simulink model "ThrottlePositionSensor"  (R2023a)
settings: Solver=FixedStepAuto  StartTime=0.0  StopTime=10.0  RelTol=1e-3
undefined symbols (not defined in the file or in its folder): TPS_Modes
libraries: pil_lib x1
settings Model: Creator=EMRIX  LastModifiedBy=EMRIX
settings OptimizationCC: DefaultParameterBehavior=Inlined  UseDivisionForNetSlopeComputation=on  GainParamInheritBuiltInType=on  UseFloatMulNetSlope=on  InlineInvariantSignals=on  PassReuseOutputArgsAs=Individual arguments  ZeroExternalMemoryAtStartup=off  ZeroInternalMemoryAtStartup=off  NoFixptDivByZeroProtection=on  EfficientFloat2IntCast=on  LifeSpan=1  OptimizeBlockOrder=speed  DifferentSizesBufferReuse=on  EfficientTunableParamExpr=on
settings DebuggingCC: ParameterTunabilityLossMsg=error
settings HardwareCC: ProdLongLongMode=on
settings SFSimCC: MATLABDynamicMemAlloc=off
settings RTWCC: Description=Embedded Coder  SystemTargetFile=ert.tlc  TemplateMakefile=ert_default_tmf  CreateSILPILBlock=SIL
settings CodeAppCC: ForceParamTrailComments=on  IgnoreCustomStorageClasses=off  OperatorAnnotations=on  SimulinkDataObjDesc=on  SFDataObjDesc=on  CustomSymbolStrGlobalVar=rt$N$M  CustomSymbolStrType=$N$M  CustomSymbolStrFcn=$N$M$F  CustomSymbolStrMacro=$N$M  InsertBlockDesc=on
settings ERTTargetCC: TargetLangStandard=C99 (ISO)  GenerateSampleERTMain=on  IncludeMdlTerminateFcn=off  CombineSignalStateStructs=on  SuppressErrorStatus=on  SupportAbsoluteTime=off  SupportComplex=off  InlinedParameterPlacement=NonHierarchical  ERTCustomFileTemplate=example_file_process.tlc  ERTFilePackagingFormat=CompactWithDataFile

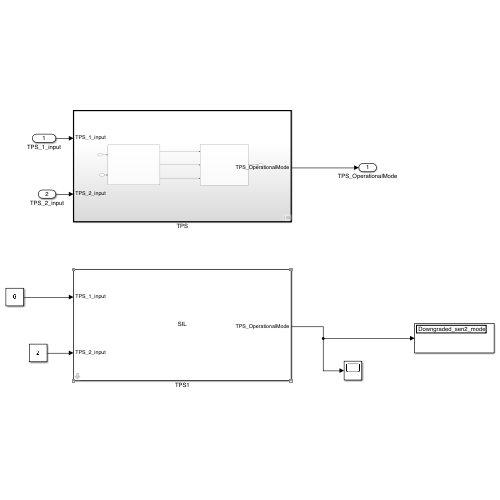
[thumbnail: Simulink's stored preview of the top-level diagram]
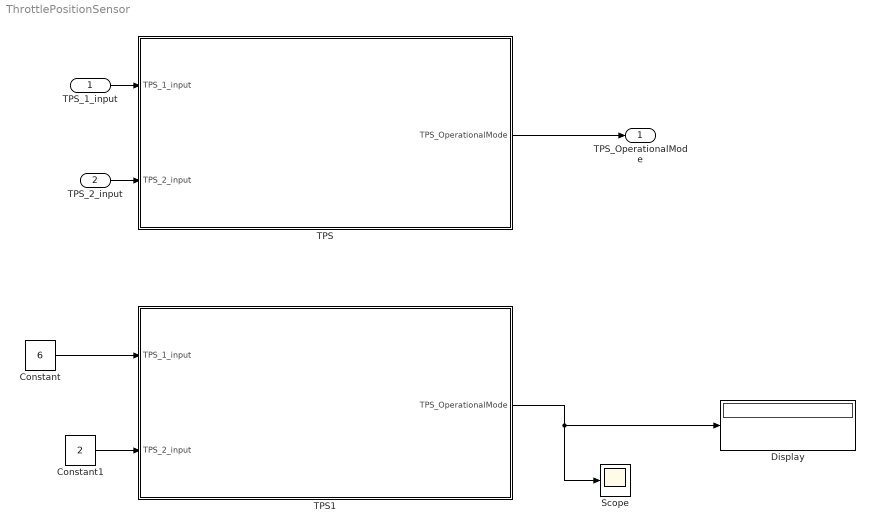
== system ThrottlePositionSensor ==
  TPS_1_input : Inport
  TPS_2_input : Inport  Port=2
  Constant : Constant  Value=6  OutDataTypeStr=Inherit: Inherit via back propagation
  Constant1 : Constant  Value=2  OutDataTypeStr=Inherit: Inherit via back propagation
  Display : Display
  Scope : Scope
  TPS : Subsystem  TreatAsAtomicUnit=on
  TPS1 : Subsystem  Tag=__SL_testing_harness_stub_  DialogController=pil_create_dialog  LoadFcn=|
      | try
      |    if ~strcmp(rtw.pil.getPILVersion, '9.14 (R2023a)_15')
      |       set_param(gcb, 'DialogController', '');
      |       set_param(gcb, 'DialogControllerArgs', '');
      |    end
      | catch e
      |       set_param(gcb, 'DialogController', '');
      |       set_param(gcb, 'DialogControllerArgs', '');
      | end
      mask help: PIL:pil:XILBlockMaskDesc
      mask Display: disp('SIL');
  TPS_OperationalMode : Outport
  wires:
  TPS/1(TPS_OperationalMode) -> TPS_OperationalMode/1
  TPS_2_input/1 -> TPS/2(TPS_2_input)
  TPS_1_input/1 -> TPS/1(TPS_1_input)
  Constant1/1 -> TPS1/2(TPS_2_input)
  Constant/1 -> TPS1/1(TPS_1_input)
  TPS1/1(TPS_OperationalMode) -> Scope/1, Display/1

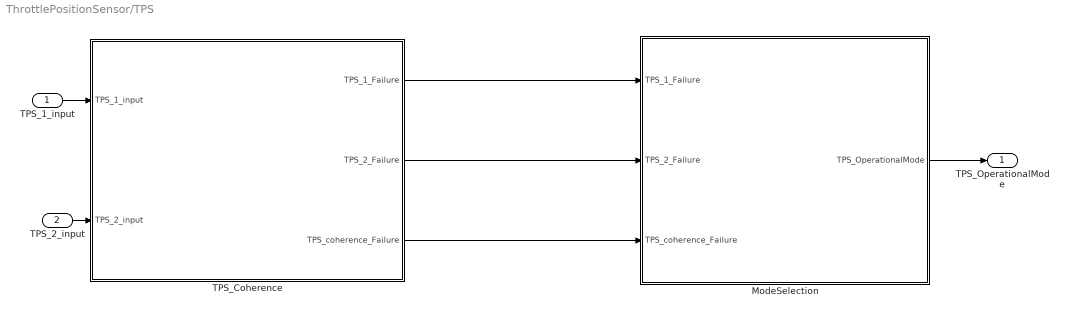
== system ThrottlePositionSensor/TPS ==
  TPS_1_input : Inport  OutDataTypeStr=single
  TPS_2_input : Inport  Port=2  OutDataTypeStr=single
  ModeSelection : Subsystem
  TPS_Coherence : Subsystem
      mask DialogControl TPS_Coherence Prompt: Parameters
  TPS_OperationalMode : Outport
  wires:
  TPS_2_input/1 -> TPS_Coherence/2(TPS_2_input)
  TPS_1_input/1 -> TPS_Coherence/1(TPS_1_input)
  ModeSelection/1(TPS_OperationalMode) -> TPS_OperationalMode/1
  TPS_Coherence/1(TPS_1_Failure) -> ModeSelection/1(TPS_1_Failure)
  TPS_Coherence/2(TPS_2_Failure) -> ModeSelection/2(TPS_2_Failure)
  TPS_Coherence/3(TPS_coherence_Failure) -> ModeSelection/3(TPS_coherence_Failure)

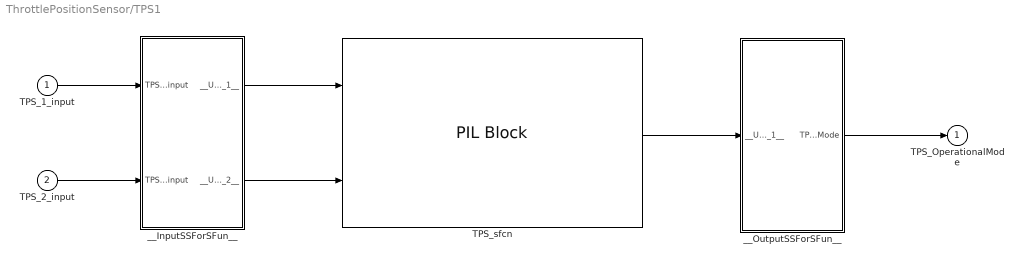
== system ThrottlePositionSensor/TPS1 ==
  TPS_1_input : Inport  OutDataTypeStr=single
  TPS_2_input : Inport  Port=2  OutDataTypeStr=single
  TPS_sfcn : pil_lib/PIL Block  SimulationMode=SIL  IsTopModelPIL=off  CodeDir=TPS_ert_rtw  AnchorDir=F:\XELLED\OS-Academy MBD\Labs\SimuLink Labs\System_Modelling_Module\TPS  ConfigName=Software-in-the-Loop (SIL)  XrelIsTopModelCode=on  XrelIsReusable=off  XrelDWorkNames={}  XrelDWorkTypes={}  XrelModelArgVals={}  XrelOrderedParamNames={}
  __InputSSForSFun__ : Subsystem
  __OutputSSForSFun__ : Subsystem
  TPS_OperationalMode : Outport
  wires:
  __OutputSSForSFun__/1(TPS_OperationalMode) -> TPS_OperationalMode/1
  TPS_sfcn/1 -> __OutputSSForSFun__/1(__UniqueInportName__1__)
  __InputSSForSFun__/2(__UniqueOutportName__2__) -> TPS_sfcn/2
  __InputSSForSFun__/1(__UniqueOutportName__1__) -> TPS_sfcn/1
  TPS_2_input/1 -> __InputSSForSFun__/2(TPS_2_input)
  TPS_1_input/1 -> __InputSSForSFun__/1(TPS_1_input)

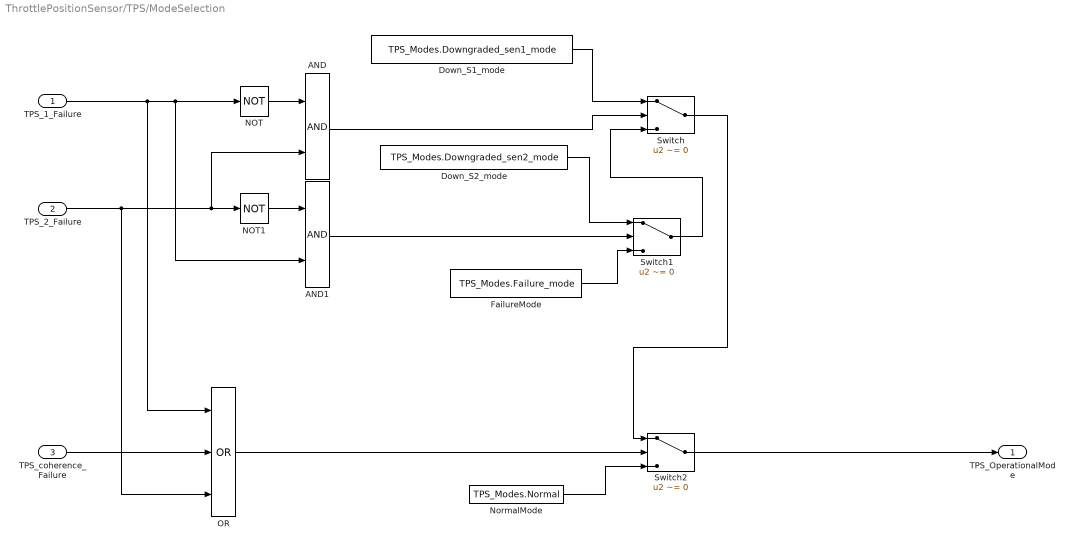
== system ThrottlePositionSensor/TPS/ModeSelection ==
  TPS_1_Failure : Inport  OutDataTypeStr=boolean
  TPS_2_Failure : Inport  Port=2  OutDataTypeStr=boolean
  TPS_coherence_Failure : Inport  Port=3  OutDataTypeStr=boolean
  AND : Logic  AllPortsSameDT=off  OutDataTypeStr=boolean
  AND1 : Logic  AllPortsSameDT=off  OutDataTypeStr=boolean
  Down_S1_mode : Constant  Value=TPS_Modes.Downgraded_sen1_mode
  Down_S2_mode : Constant  Value=TPS_Modes.Downgraded_sen2_mode
  FailureMode : Constant  Value=TPS_Modes.Failure_mode
  NOT : Logic  Operator=NOT  AllPortsSameDT=off  OutDataTypeStr=boolean
  NOT1 : Logic  Operator=NOT  AllPortsSameDT=off  OutDataTypeStr=boolean
  NormalMode : Constant  Value=TPS_Modes.Normal
  OR : Logic  Operator=OR  Inputs=3  AllPortsSameDT=off  OutDataTypeStr=boolean
  Switch : Switch  Criteria=u2 ~= 0  SaturateOnIntegerOverflow=off  InputSameDT=off
  Switch1 : Switch  Criteria=u2 ~= 0  SaturateOnIntegerOverflow=off  InputSameDT=off
  Switch2 : Switch  Criteria=u2 ~= 0  SaturateOnIntegerOverflow=off  InputSameDT=off
  TPS_OperationalMode : Outport
  wires:
  NOT/1 -> AND/1
  AND/1 -> Switch/2
  TPS_1_Failure/1 -> OR/1, NOT/1, AND1/2
  AND1/1 -> Switch1/2
  TPS_2_Failure/1 -> OR/3, AND/2, NOT1/1
  NOT1/1 -> AND1/1
  Down_S1_mode/1 -> Switch/1
  Switch1/1 -> Switch/3
  Down_S2_mode/1 -> Switch1/1
  Switch/1 -> Switch2/1
  NormalMode/1 -> Switch2/3
  FailureMode/1 -> Switch1/3
  Switch2/1 -> TPS_OperationalMode/1
  TPS_coherence_Failure/1 -> OR/2
  OR/1 -> Switch2/2

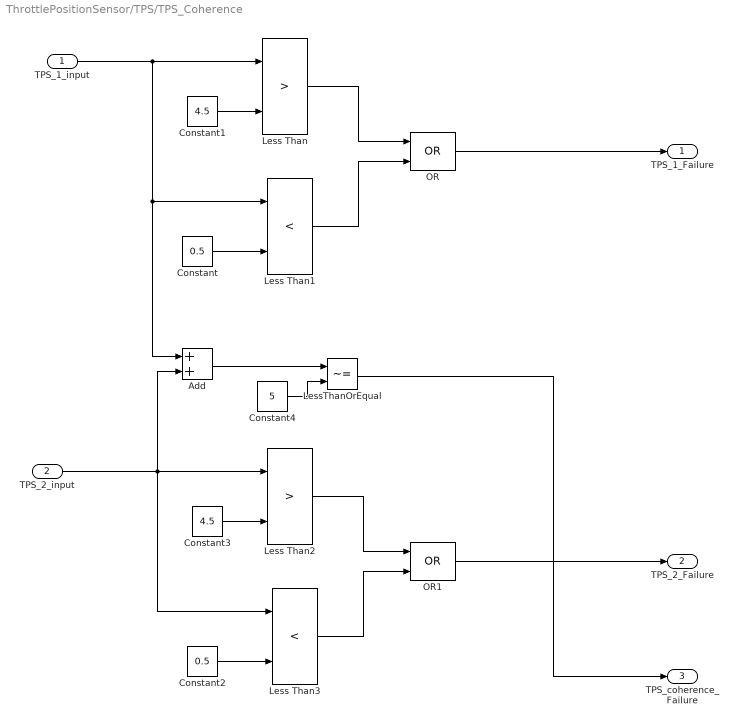
== system ThrottlePositionSensor/TPS/TPS_Coherence ==
  TPS_1_input : Inport  OutDataTypeStr=single
  TPS_2_input : Inport  Port=2  OutDataTypeStr=single
  Add : Sum
  Constant : Constant  Value=0.5
  Constant1 : Constant  Value=4.5
  Constant2 : Constant  Value=0.5
  Constant3 : Constant  Value=4.5
  Constant4 : Constant  Value=5
  Less Than : RelationalOperator  Operator=>  OutDataTypeStr=boolean  RndMeth=Simplest  InputSameDT=off
  Less Than1 : RelationalOperator  Operator=<  OutDataTypeStr=boolean  RndMeth=Simplest  InputSameDT=off
  Less Than2 : RelationalOperator  Operator=>  OutDataTypeStr=boolean  RndMeth=Simplest  InputSameDT=off
  Less Than3 : RelationalOperator  Operator=<  OutDataTypeStr=boolean  RndMeth=Simplest  InputSameDT=off
  LessThanOrEqual : RelationalOperator  Operator=~=  OutDataTypeStr=boolean  RndMeth=Simplest  InputSameDT=off
  OR : Logic  Operator=OR  IconShape=distinctive  AllPortsSameDT=off  OutDataTypeStr=boolean
  OR1 : Logic  Operator=OR  IconShape=distinctive  AllPortsSameDT=off  OutDataTypeStr=boolean
  TPS_1_Failure : Outport  OutDataTypeStr=boolean
  TPS_2_Failure : Outport  Port=2  OutDataTypeStr=boolean
  TPS_coherence_Failure : Outport  Port=3  OutDataTypeStr=boolean
  wires:
  TPS_1_input/1 -> Add/1, Less Than1/1, Less Than/1
  Constant3/1 -> Less Than2/2
  Less Than1/1 -> OR/2
  Constant1/1 -> Less Than/2
  OR/1 -> TPS_1_Failure/1
  Constant/1 -> Less Than1/2
  Constant4/1 -> LessThanOrEqual/2
  Less Than/1 -> OR/1
  TPS_2_input/1 -> Less Than3/1, Add/2, Less Than2/1
  Less Than3/1 -> OR1/2
  Add/1 -> LessThanOrEqual/1
  Less Than2/1 -> OR1/1
  LessThanOrEqual/1 -> TPS_coherence_Failure/1
  OR1/1 -> TPS_2_Failure/1
  Constant2/1 -> Less Than3/2

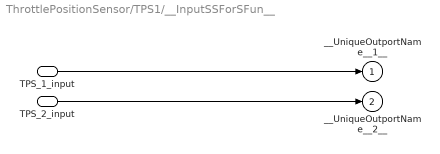
== system ThrottlePositionSensor/TPS1/__InputSSForSFun__ ==
  TPS_1_input : Inport  OutDataTypeStr=single
  TPS_2_input : Inport  Port=2  OutDataTypeStr=single
  __UniqueOutportName__1__ : Outport
  __UniqueOutportName__2__ : Outport  Port=2
  wires:
  TPS_2_input/1 -> __UniqueOutportName__2__/1
  TPS_1_input/1 -> __UniqueOutportName__1__/1

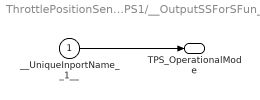
== system ThrottlePositionSensor/TPS1/__OutputSSForSFun__ ==
  __UniqueInportName__1__ : Inport
  TPS_OperationalMode : Outport
  wires:
  __UniqueInportName__1__/1 -> TPS_OperationalMode/1
